simulink model "ssp4"  (R2014a)
settings: Solver=ode45  StartTime=0.0  StopTime=5  RelTol=1e-3
libraries: dspvision x2
settings Model: SimulationMode=accelerator  Creator=root  LastModifiedBy=root

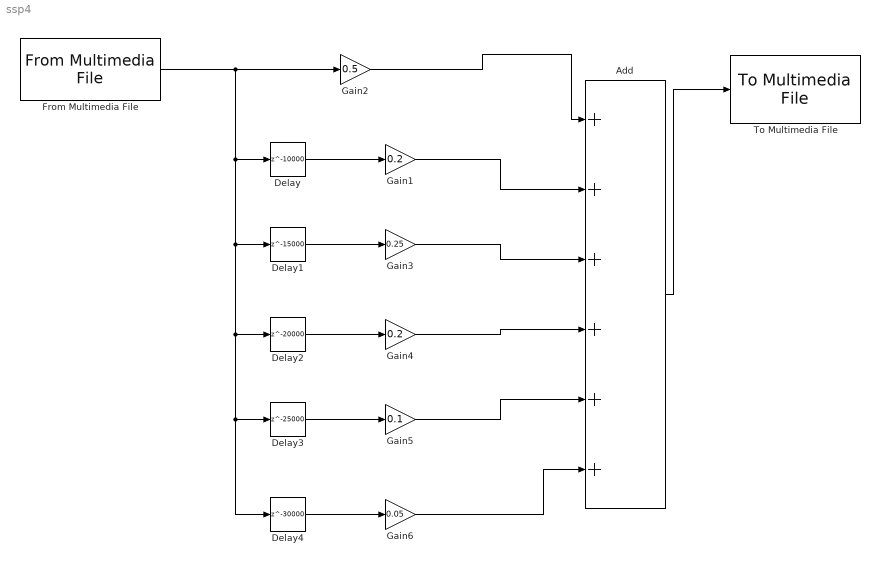
== system ssp4 ==
  Add : Sum  Inputs=++++++
  Delay : Delay  DelayLength=10000  InitialCondition=0
  Delay1 : Delay  DelayLength=15000  InitialCondition=0
  Delay2 : Delay  DelayLength=20000  InitialCondition=0
  Delay3 : Delay  DelayLength=25000  InitialCondition=0
  Delay4 : Delay  DelayLength=30000  InitialCondition=0
  From Multimedia File : dspvision/From Multimedia File  inputFilename=/home/brjathu/Desktop/speech_dft.wav  loop=on  numPlays=inf  outputStreams=Audio only  videoDataType=int16  audioDataType=int16  inheritSampleTime=on  userDefinedSampleTime=1/30  noAudioOutput=off  isIntensityVideo=off  fourcc=RGB  colorVideoFormat=One multidimensional signal  outputEOF=off  dataOrg=Column-major  audioFrameSize=1  computeAudioFrameSize=off  outSamplingMode=Sample based
  Gain1 : Gain  Gain=0.2  OutDataTypeStr=int16
  Gain2 : Gain  Gain=0.5  OutDataTypeStr=int16
  Gain3 : Gain  Gain=0.25  OutDataTypeStr=int16
  Gain4 : Gain  Gain=0.2  OutDataTypeStr=int16
  Gain5 : Gain  Gain=0.1  OutDataTypeStr=int16
  Gain6 : Gain  Gain=0.05  OutDataTypeStr=int16
  To Multimedia File : dspvision/To Multimedia File  outputFilename=output.wav  streamSelection=Audio only  videoCompressor=None (uncompressed)  audioCompressor=None (uncompressed)  imagePorts=One multidimensional signal  fileType=WAV  audioDatatype=Determine from input data type  fourcc=RGB  videoQuality=75  mj2000CompFactor=10
  wires:
  Delay/1 -> Gain1/1
  Gain2/1 -> Add/1
  Gain1/1 -> Add/2
  Add/1 -> To Multimedia File/1
  Delay1/1 -> Gain3/1
  Gain3/1 -> Add/3
  Delay2/1 -> Gain4/1
  Gain4/1 -> Add/4
  Delay3/1 -> Gain5/1
  Gain5/1 -> Add/5
  From Multimedia File/1 -> Gain2/1, Delay4/1, Delay3/1, Delay2/1, Delay1/1, Delay/1
  Delay4/1 -> Gain6/1
  Gain6/1 -> Add/6
